simulink model "VehicleDynamicsModel"  (R2016b)
settings: Solver=VariableStepAuto  StartTime=0.0  StopTime=50  RelTol=1e-3
libraries: simulink x1
settings Model: Creator=shangguanlantian  LastModifiedBy=shangguanlantian

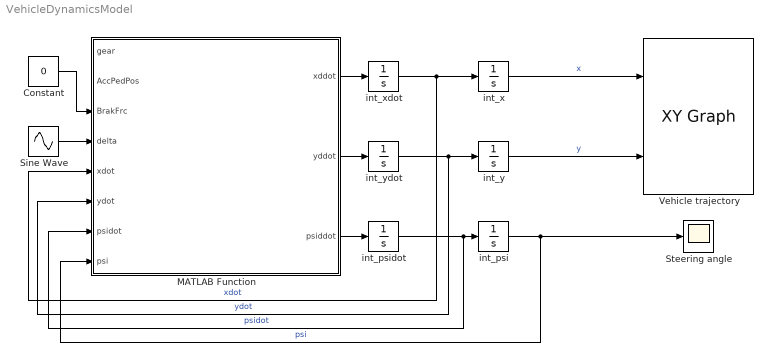
== system VehicleDynamicsModel ==
  Constant : Constant  Value=0
  MATLAB Function : MATLAB Function  TreatAsAtomicUnit=on
  Sine Wave : Sin  SampleTime=0
  Steering angle : Scope
  Vehicle trajectory : simulink/Sinks/XY Graph  xmin=-1  xmax=100  ymin=-1  ymax=100  st=-1
  int_psi : Integrator
  int_psidot : Integrator  InitialCondition=1
  int_x : Integrator
  int_xdot : Integrator  InitialCondition=1
  int_y : Integrator
  int_ydot : Integrator  InitialCondition=1
  wires:
  MATLAB Function/1(xddot) -> int_xdot/1
  MATLAB Function/2(yddot) -> int_ydot/1
  MATLAB Function/3(psiddot) -> int_psidot/1
  int_xdot/1 -> MATLAB Function/5(xdot), int_x/1  "xdot"
  int_ydot/1 -> MATLAB Function/6(ydot), int_y/1  "ydot"
  int_psidot/1 -> MATLAB Function/7(psidot), int_psi/1  "psidot"
  int_x/1 -> Vehicle trajectory/1  "x"
  int_y/1 -> Vehicle trajectory/2  "y"
  int_psi/1 -> Steering angle/1, MATLAB Function/8(psi)  "psi"
  Sine Wave/1 -> MATLAB Function/4(delta)
  Constant/1 -> MATLAB Function/3(BrakFrc)

== matlab function VehicleDynamicsModel/MATLAB Function ==
  data: gear input; AccPedPos input; BrakFrc input; xddot output; delta input; xdot input; ydot input; psidot input; psi input; yddot output; psiddot output
function [xddot,yddot,psiddot] = VDM4dof(gear,AccPedPos,BrakFrc,delta,xdot,ydot,psidot,psi)
% For simplicity, tractive effort is estimated without calculating using gear number and acceleration pedal position
FB = BrakFrc;
% parameters:
m = 1239; % [kg] car mass
g = 9.81; % [m/s^2] gravitational acceleration
lv = 1.19016; % [m] distance between CoG and front wheel
lh = 1.37484; % [m] distance between CoG and rear wheel
eSP = 0.5; % [m] distance between CoG and drag mount point
R = 0.302; % [m] wheel radius
Izz = 1752; % [kgm^2] moment of inertia
% iL = 21.1; % steering wheel transmission
% IR = 1.5; % moment of inertia of wheel
comega = 0.3; % air drag coefficient
rho = 1.249512; % [N/m^2] air density
A = 1.4378946874; % [m^2] effective flow surface
cy = 0.3; % lateral air drag coefficient
cAT1v = 3317.99; % tyre coefficient AT-model
cAT1h = 2872.99; % tyre coefficient AT-model
cAT2v = 30; % tyre coefficient AT-model
cAT2h = 30; % tyre coefficient AT-model
fR0 = 0.009; % rolling resistance coefficient
fR1 = 0.002; % rolling resistance coefficient
fR4 = 0.0003; % rolling resistance coefficient
Fte = 200000; % [N] estimated tractive effort
% velocity amplitude:
v = (xdot^2+ydot^2)^(0.5);
% slip angle of body:
beta = psi-atan(ydot/xdot);
% slip angles of wheels:
alphav = delta-atan((lv*psidot-v*sin(beta))/(v*cos(beta)));
alphah = atan((lh*psidot+v*sin(beta))/(v*cos(beta)));
% braking force controlled by driver:
FBv = 2/3*FB;
FBh = 1/3*FB;
% friction coefficient:
fRv = fR0+fR1*v/100+fR4*(v/100)^2;
% static tyre loads:
Fzv = (m*lh*g)/(lv+lh);
Fzh = (m*lv*g)/(lv+lh);
% rolling resistance force:
FRv = fRv*Fzv;
FRh = fRv*Fzh;
% longitudinal forces:
Fuv = -FBv-FRv;
Fuh = Fte-FBh-FRh; % Fuh = (Mwheel/R)-FBh-FRh;
% lateral tyre forces:
Fsv = cAT1v*atan(cAT2v*alphav);
Fsh = cAT1h*atan(cAT2h*alphah);
% air resistance:
Flx = 0.5*comega*rho*A*(v^2);
Fly = 0.5*cy*rho*A*(v*R^2);

% equations of motion:
xddot = (1/m)*((Fuh-Flx)*cos(psi)+Fuv*cos(delta+psi)-Fsv*sin(delta+psi)-(Fsh-Fly)*sin(psi));
yddot = (1/m)*((Fuh-Flx)*sin(psi)+Fuv*sin(delta+psi)+Fsv*cos(delta+psi)+(Fsh-Fly)*cos(psi));
psiddot = (1/Izz)*(Fsv*lv*cos(delta)-Fsh*lh-Fly*eSP+Fuv*lv*sin(delta));
